simulink model "simulink"  (R2015a)
settings: Solver=ode4  StartTime=0.0  StopTime=inf  FixedStep=1e-3  RelTol=1e-3
values from neighbouring files (symbols this model uses):
  b_end1 = 0.5*(k_end1*Cyl1.m)^0.5    [m-script.m]
  b_end2 = 0.5*(k_end2*Cyl2.m)^0.5    [m-script.m]
  b_end3 = 0.5*(k_end3*Cyl3.m)^0.5    [m-script.m]
  b_end4 = 0.5*(k_end4*Cyl4.m)^0.5    [m-script.m]
  Cyl1_b = 40000    [m-script.m]
  Cyl1_Fc = 20514    [m-script.m]
  Cyl1_Fs = 22360    [m-script.m]
  Cyl1_K = 20000    [m-script.m]
  Cyl1_vs = 0.8    [m-script.m]
  Cyl2_b = 30000    [m-script.m]
  Cyl2_Fc = 14950    [m-script.m]
  Cyl2_Fs = 16125    [m-script.m]
  Cyl2_K = 20000    [m-script.m]
  Cyl2_vs = 0.8    [m-script.m]
  Cyl3_b = 30000    [m-script.m]
  Cyl3_Fc = 14996    [m-script.m]
  Cyl3_Fs = 16340    [m-script.m]
  Cyl3_K = 20000    [m-script.m]
  Cyl3_vs = 0.8    [m-script.m]
  Cyl4_b = 8500    [m-script.m]
  Cyl4_Fc = 4570    [m-script.m]
  Cyl4_Fs = 4945    [m-script.m]
  Cyl4_K = 20000    [m-script.m]
  Cyl4_vs = 0.8    [m-script.m]
  k_end1 = (pr_Ps*Cyl1.A_A)/v1    [m-script.m]
  k_end2 = (pr_Ps*Cyl2.A_A)/v2    [m-script.m]
  k_end3 = (pr_Ps*Cyl3.A_A)/v3    [m-script.m]
  k_end4 = (pr_Ps*Cyl4.A_A)/v4    [m-script.m]
  pr_Ps = 215e5    (= 21500000)    [m-script.m]
  sampleTime = 0.001    [m-script.m]
  Valve_eta = 0.989    [m-script.m]
  Valve_omega = 40.5    [m-script.m]
undefined symbols (not defined in the file or in its folder): Cyl, Cyl1, Cyl2, Cyl3, Cyl4, Cylinder2, Cylinder3, Cylinder4, Extention1, Extention2, Lift, Link1, Pillar, Pinion, Piston2, Piston3, Piston4, Rack, Tilt, Valve, X, Y, Z
undefined symbols (not defined in the file): Valve1, Valve2, Valve3, Valve4
libraries: sm_lib x72, simulink x32, nesl_utility x20, simulink_extras x3, xpcrtudplib x2, xpcobsoletelib x2
(part 4 of 4)

== system simulink/Hydraulics/Cylinder 5/Cylinder/Chamber A ==
  Q_in : Inport
  " dv_A/dt" : Inport  Port=2
  " V_A" : Inport  Port=3
  " B" : Inport  Port=4
  Integrator : Integrator  InitialCondition=pinitial  AbsoluteTolerance=10
  Product : Product  Inputs=*/*  SaturateOnIntegerOverflow=on  InputSameDT=on  OutDataTypeStr=Inherit: Same as first input
  Saturation : Saturate  UpperLimit=inf  LowerLimit=0
  Sum : Sum  Inputs=+-  SaturateOnIntegerOverflow=on  InputSameDT=on  OutDataTypeStr=Inherit: Same as first input
  p_A : Outport
  wires:
  " V_A"/1 -> Product/2
  " dv_A/dt"/1 -> Sum/2
  Product/1 -> Integrator/1
  Integrator/1 -> Saturation/1
  Saturation/1 -> p_A/1
  " B"/1 -> Product/3
  Q_in/1 -> Sum/1
  Sum/1 -> Product/1

== system simulink/Hydraulics/Cylinder 5/Cylinder/Chamber B ==
  B : Inport
  V_B : Inport  Port=2
  dv_B/dt : Inport  Port=3
  Q_in : Inport  Port=4
  Integrator : Integrator  InitialCondition=pinitial  AbsoluteTolerance=10
  Product : Product  Inputs=*/*  SaturateOnIntegerOverflow=on  InputSameDT=on  OutDataTypeStr=Inherit: Same as first input
  Saturation : Saturate  UpperLimit=inf  LowerLimit=0
  Sum : Sum  Inputs=+-  SaturateOnIntegerOverflow=on  InputSameDT=on  OutDataTypeStr=Inherit: Same as first input
  p_B : Outport
  wires:
  V_B/1 -> Product/2
  dv_B/dt/1 -> Sum/2
  Sum/1 -> Product/1
  Q_in/1 -> Sum/1
  B/1 -> Product/3
  Saturation/1 -> p_B/1
  Integrator/1 -> Saturation/1
  Product/1 -> Integrator/1

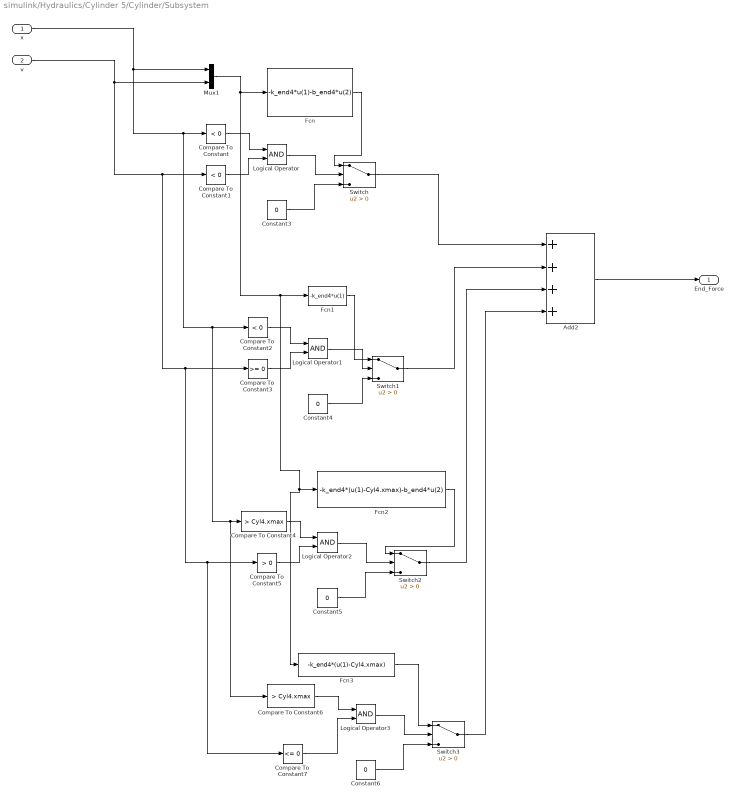
== system simulink/Hydraulics/Cylinder 5/Cylinder/Subsystem ==
  x : Inport
  v : Inport  Port=2
  Add2 : Sum  Inputs=++++
  Compare To Constant : simulink/Logic and Bit Operations/Compare To Constant  relop=<  const=0  OutDataTypeStr=boolean
  Compare To Constant1 : simulink/Logic and Bit Operations/Compare To Constant  relop=<  const=0  OutDataTypeStr=boolean
  Compare To Constant2 : simulink/Logic and Bit Operations/Compare To Constant  relop=<  const=0  OutDataTypeStr=boolean
  Compare To Constant3 : simulink/Logic and Bit Operations/Compare To Constant  relop=>=  const=0  OutDataTypeStr=boolean
  Compare To Constant4 : simulink/Logic and Bit Operations/Compare To Constant  relop=>  const=Cyl4.xmax  OutDataTypeStr=boolean
  Compare To Constant5 : simulink/Logic and Bit Operations/Compare To Constant  relop=>  const=0  OutDataTypeStr=boolean
  Compare To Constant6 : simulink/Logic and Bit Operations/Compare To Constant  relop=>  const=Cyl4.xmax  OutDataTypeStr=boolean
  Compare To Constant7 : simulink/Logic and Bit Operations/Compare To Constant  relop=<=  const=0  OutDataTypeStr=boolean
  Constant{3..6} (4 alike) : Constant  Value=0
  Fcn : Fcn  Expr=-k_end4*u(1)-b_end4*u(2)
  Fcn1 : Fcn  Expr=-k_end4*u(1)
  Fcn2 : Fcn  Expr=-k_end4*(u(1)-Cyl4.xmax)-b_end4*u(2)
  Fcn3 : Fcn  Expr=-k_end4*(u(1)-Cyl4.xmax)
  Logical Operator{,1..3} (4 alike) : Logic  AllPortsSameDT=off  OutDataTypeStr=boolean
  Mux1 : Mux  Inputs=2
  Switch{,1..3} (4 alike) : Switch  Criteria=u2 > Threshold
  End_Force : Outport
  wires:
  x/1 -> Compare To Constant/1, Compare To Constant2/1, Compare To Constant6/1, Compare To Constant4/1, Mux1/1
  v/1 -> Mux1/2, Compare To Constant1/1, Compare To Constant3/1, Compare To Constant5/1, Compare To Constant7/1
  Fcn2/1 -> Switch2/1
  Logical Operator3/1 -> Switch3/2
  Fcn3/1 -> Switch3/1
  Compare To Constant5/1 -> Logical Operator2/2
  Constant6/1 -> Switch3/3
  Switch2/1 -> Add2/3
  Compare To Constant6/1 -> Logical Operator3/1
  Switch/1 -> Add2/1
  Logical Operator2/1 -> Switch2/2
  Compare To Constant7/1 -> Logical Operator3/2
  Switch1/1 -> Add2/2
  Add2/1 -> End_Force/1
  Mux1/1 -> Fcn1/1, Fcn2/1, Fcn3/1, Fcn/1
  Switch3/1 -> Add2/4
  Compare To Constant2/1 -> Logical Operator1/1
  Compare To Constant1/1 -> Logical Operator/2
  Constant5/1 -> Switch2/3
  Constant4/1 -> Switch1/3
  Logical Operator1/1 -> Switch1/2
  Fcn/1 -> Switch/1
  Logical Operator/1 -> Switch/2
  Constant3/1 -> Switch/3
  Compare To Constant/1 -> Logical Operator/1
  Compare To Constant4/1 -> Logical Operator2/1
  Fcn1/1 -> Switch1/1
  Compare To Constant3/1 -> Logical Operator1/2

== system simulink/Hydraulics/Cylinder 1/4//3 Valve/Flow paths/Orifice AT ==
  p_A : Inport
  p_T : Inport  Port=2
  u : Inport  Port=3
  Abs : Abs  ZeroCross=off  SaturateOnIntegerOverflow=on
  Add : Sum  Inputs=+-
  Fcn : Fcn  Expr=u[2]*u[1]/2.0/sqrt(ptr)*(3-u[1]/ptr)
  Fcn-Saturation : Fcn  Expr=(u(1)>=-1e-10)*u(1)
  Gain : Gain  Gain=K  SaturateOnIntegerOverflow=on  OutDataTypeStr=Inherit: Same as input  ParamDataTypeStr=Inherit: Same as input
  Gain1 : Gain  Gain=-1  SaturateOnIntegerOverflow=on  OutDataTypeStr=Inherit: Same as input  ParamDataTypeStr=Inherit: Same as input
  Math Function1 : Math  Operator=sqrt  SaturateOnIntegerOverflow=on
  Mux : Mux  Inputs=2
  Product : Product  SaturateOnIntegerOverflow=on  InputSameDT=on  OutDataTypeStr=Inherit: Same as first input
  Product1 : Product  SaturateOnIntegerOverflow=on  InputSameDT=on  OutDataTypeStr=Inherit: Same as first input
  Sign : Signum  ZeroCross=off
  "Switch, treshold = ptr" : Switch  Threshold=ptr  ZeroCross=off  SaturateOnIntegerOverflow=on
  Q_A : Outport  InitialOutput=0
  Q_T : Outport  Port=2  InitialOutput=0
  wires:
  u/1 -> Fcn-Saturation/1
  Fcn/1 -> "Switch, treshold = ptr"/3
  Mux/1 -> Fcn/1
  Product/1 -> "Switch, treshold = ptr"/1
  Math Function1/1 -> Product/1
  Abs/1 -> "Switch, treshold = ptr"/2, Mux/1, Math Function1/1
  Fcn-Saturation/1 -> Gain/1
  Gain/1 -> Product/2, Mux/2
  "Switch, treshold = ptr"/1 -> Product1/2
  Sign/1 -> Product1/1
  p_A/1 -> Add/1
  p_T/1 -> Add/2
  Add/1 -> Abs/1, Sign/1
  Product1/1 -> Q_T/1, Gain1/1
  Gain1/1 -> Q_A/1

== system simulink/Hydraulics/Cylinder 1/4//3 Valve/Flow paths/Orifice BT ==
  p_T : Inport
  p_B : Inport  Port=2
  u : Inport  Port=3
  Abs : Abs  ZeroCross=off  SaturateOnIntegerOverflow=on
  Add : Sum  Inputs=+-
  Fcn : Fcn  Expr=u[2]*u[1]/2.0/sqrt(ptr)*(3-u[1]/ptr)
  Fcn-Saturation : Fcn  Expr=(u(1)>=-1e-10)*u(1)
  Gain : Gain  Gain=K  SaturateOnIntegerOverflow=on  OutDataTypeStr=Inherit: Same as input  ParamDataTypeStr=Inherit: Same as input
  Gain1 : Gain  Gain=-1  SaturateOnIntegerOverflow=on  OutDataTypeStr=Inherit: Same as input  ParamDataTypeStr=Inherit: Same as input
  Math Function1 : Math  Operator=sqrt  SaturateOnIntegerOverflow=on
  Mux : Mux  Inputs=2
  Product : Product  SaturateOnIntegerOverflow=on  InputSameDT=on  OutDataTypeStr=Inherit: Same as first input
  Product1 : Product  SaturateOnIntegerOverflow=on  InputSameDT=on  OutDataTypeStr=Inherit: Same as first input
  Sign : Signum  ZeroCross=off
  "Switch, treshold = ptr" : Switch  Threshold=ptr  ZeroCross=off  SaturateOnIntegerOverflow=on
  Q_T : Outport  InitialOutput=0
  Q_B : Outport  Port=2  InitialOutput=0
  wires:
  Gain1/1 -> Q_T/1
  Product1/1 -> Gain1/1, Q_B/1
  Add/1 -> Sign/1, Abs/1
  p_B/1 -> Add/2
  p_T/1 -> Add/1
  Sign/1 -> Product1/1
  "Switch, treshold = ptr"/1 -> Product1/2
  Gain/1 -> Mux/2, Product/2
  Fcn-Saturation/1 -> Gain/1
  Abs/1 -> Math Function1/1, Mux/1, "Switch, treshold = ptr"/2
  Math Function1/1 -> Product/1
  Product/1 -> "Switch, treshold = ptr"/1
  Mux/1 -> Fcn/1
  Fcn/1 -> "Switch, treshold = ptr"/3
  u/1 -> Fcn-Saturation/1

== system simulink/Hydraulics/Cylinder 1/4//3 Valve/Flow paths/Orifice PA ==
  p_P : Inport
  p_A : Inport  Port=2
  u : Inport  Port=3
  Abs : Abs  ZeroCross=off  SaturateOnIntegerOverflow=on
  Add : Sum  Inputs=+-
  Fcn : Fcn  Expr=u[2]*u[1]/2.0/sqrt(ptr)*(3-u[1]/ptr)
  Fcn-Saturation : Fcn  Expr=(u(1)>=-1e-10)*u(1)
  Gain : Gain  Gain=K  SaturateOnIntegerOverflow=on  OutDataTypeStr=Inherit: Same as input  ParamDataTypeStr=Inherit: Same as input
  Gain1 : Gain  Gain=-1  SaturateOnIntegerOverflow=on  OutDataTypeStr=Inherit: Same as input  ParamDataTypeStr=Inherit: Same as input
  Math Function1 : Math  Operator=sqrt  SaturateOnIntegerOverflow=on
  Mux : Mux  Inputs=2
  Product : Product  SaturateOnIntegerOverflow=on  InputSameDT=on  OutDataTypeStr=Inherit: Same as first input
  Product1 : Product  SaturateOnIntegerOverflow=on  InputSameDT=on  OutDataTypeStr=Inherit: Same as first input
  Sign : Signum  ZeroCross=off
  "Switch, treshold = ptr" : Switch  Threshold=ptr  ZeroCross=off  SaturateOnIntegerOverflow=on
  Q_P : Outport  InitialOutput=0
  Q_A : Outport  Port=2  InitialOutput=0
  wires:
  u/1 -> Fcn-Saturation/1
  Fcn/1 -> "Switch, treshold = ptr"/3
  Mux/1 -> Fcn/1
  Product/1 -> "Switch, treshold = ptr"/1
  Math Function1/1 -> Product/1
  Abs/1 -> "Switch, treshold = ptr"/2, Mux/1, Math Function1/1
  Fcn-Saturation/1 -> Gain/1
  Gain/1 -> Product/2, Mux/2
  "Switch, treshold = ptr"/1 -> Product1/2
  Sign/1 -> Product1/1
  p_P/1 -> Add/1
  p_A/1 -> Add/2
  Add/1 -> Abs/1, Sign/1
  Product1/1 -> Q_A/1, Gain1/1
  Gain1/1 -> Q_P/1

== system simulink/Hydraulics/Cylinder 1/4//3 Valve/Flow paths/Orifice PB ==
  p_B : Inport
  p_P : Inport  Port=2
  u : Inport  Port=3
  Abs : Abs  ZeroCross=off  SaturateOnIntegerOverflow=on
  Add : Sum  Inputs=+-
  Fcn : Fcn  Expr=u[2]*u[1]/2.0/sqrt(ptr)*(3-u[1]/ptr)
  Fcn-Saturation : Fcn  Expr=(u(1)>=-1e-10)*u(1)
  Gain : Gain  Gain=K  SaturateOnIntegerOverflow=on  OutDataTypeStr=Inherit: Same as input  ParamDataTypeStr=Inherit: Same as input
  Gain1 : Gain  Gain=-1  SaturateOnIntegerOverflow=on  OutDataTypeStr=Inherit: Same as input  ParamDataTypeStr=Inherit: Same as input
  Math Function1 : Math  Operator=sqrt  SaturateOnIntegerOverflow=on
  Mux : Mux  Inputs=2
  Product : Product  SaturateOnIntegerOverflow=on  InputSameDT=on  OutDataTypeStr=Inherit: Same as first input
  Product1 : Product  SaturateOnIntegerOverflow=on  InputSameDT=on  OutDataTypeStr=Inherit: Same as first input
  Sign : Signum  ZeroCross=off
  "Switch, treshold = ptr" : Switch  Threshold=ptr  ZeroCross=off  SaturateOnIntegerOverflow=on
  Q_B : Outport  InitialOutput=0
  Q_P : Outport  Port=2  InitialOutput=0
  wires:
  Gain1/1 -> Q_B/1
  Product1/1 -> Gain1/1, Q_P/1
  Add/1 -> Sign/1, Abs/1
  p_P/1 -> Add/2
  p_B/1 -> Add/1
  Sign/1 -> Product1/1
  "Switch, treshold = ptr"/1 -> Product1/2
  Gain/1 -> Mux/2, Product/2
  Fcn-Saturation/1 -> Gain/1
  Abs/1 -> Math Function1/1, Mux/1, "Switch, treshold = ptr"/2
  Math Function1/1 -> Product/1
  Product/1 -> "Switch, treshold = ptr"/1
  Mux/1 -> Fcn/1
  Fcn/1 -> "Switch, treshold = ptr"/3
  u/1 -> Fcn-Saturation/1

== system simulink/Hydraulics/Cylinder 2/4//3 Valve/Flow paths/Orifice AT ==
  p_A : Inport
  p_T : Inport  Port=2
  u : Inport  Port=3
  Abs : Abs  ZeroCross=off  SaturateOnIntegerOverflow=on
  Add : Sum  Inputs=+-
  Fcn : Fcn  Expr=u[2]*u[1]/2.0/sqrt(ptr)*(3-u[1]/ptr)
  Fcn-Saturation : Fcn  Expr=(u(1)>=-1e-10)*u(1)
  Gain : Gain  Gain=K  SaturateOnIntegerOverflow=on  OutDataTypeStr=Inherit: Same as input  ParamDataTypeStr=Inherit: Same as input
  Gain1 : Gain  Gain=-1  SaturateOnIntegerOverflow=on  OutDataTypeStr=Inherit: Same as input  ParamDataTypeStr=Inherit: Same as input
  Math Function1 : Math  Operator=sqrt  SaturateOnIntegerOverflow=on
  Mux : Mux  Inputs=2
  Product : Product  SaturateOnIntegerOverflow=on  InputSameDT=on  OutDataTypeStr=Inherit: Same as first input
  Product1 : Product  SaturateOnIntegerOverflow=on  InputSameDT=on  OutDataTypeStr=Inherit: Same as first input
  Sign : Signum  ZeroCross=off
  "Switch, treshold = ptr" : Switch  Threshold=ptr  ZeroCross=off  SaturateOnIntegerOverflow=on
  Q_A : Outport  InitialOutput=0
  Q_T : Outport  Port=2  InitialOutput=0
  wires:
  u/1 -> Fcn-Saturation/1
  Fcn/1 -> "Switch, treshold = ptr"/3
  Mux/1 -> Fcn/1
  Product/1 -> "Switch, treshold = ptr"/1
  Math Function1/1 -> Product/1
  Abs/1 -> "Switch, treshold = ptr"/2, Mux/1, Math Function1/1
  Fcn-Saturation/1 -> Gain/1
  Gain/1 -> Product/2, Mux/2
  "Switch, treshold = ptr"/1 -> Product1/2
  Sign/1 -> Product1/1
  p_A/1 -> Add/1
  p_T/1 -> Add/2
  Add/1 -> Abs/1, Sign/1
  Product1/1 -> Q_T/1, Gain1/1
  Gain1/1 -> Q_A/1

== system simulink/Hydraulics/Cylinder 2/4//3 Valve/Flow paths/Orifice BT ==
  p_T : Inport
  p_B : Inport  Port=2
  u : Inport  Port=3
  Abs : Abs  ZeroCross=off  SaturateOnIntegerOverflow=on
  Add : Sum  Inputs=+-
  Fcn : Fcn  Expr=u[2]*u[1]/2.0/sqrt(ptr)*(3-u[1]/ptr)
  Fcn-Saturation : Fcn  Expr=(u(1)>=-1e-10)*u(1)
  Gain : Gain  Gain=K  SaturateOnIntegerOverflow=on  OutDataTypeStr=Inherit: Same as input  ParamDataTypeStr=Inherit: Same as input
  Gain1 : Gain  Gain=-1  SaturateOnIntegerOverflow=on  OutDataTypeStr=Inherit: Same as input  ParamDataTypeStr=Inherit: Same as input
  Math Function1 : Math  Operator=sqrt  SaturateOnIntegerOverflow=on
  Mux : Mux  Inputs=2
  Product : Product  SaturateOnIntegerOverflow=on  InputSameDT=on  OutDataTypeStr=Inherit: Same as first input
  Product1 : Product  SaturateOnIntegerOverflow=on  InputSameDT=on  OutDataTypeStr=Inherit: Same as first input
  Sign : Signum  ZeroCross=off
  "Switch, treshold = ptr" : Switch  Threshold=ptr  ZeroCross=off  SaturateOnIntegerOverflow=on
  Q_T : Outport  InitialOutput=0
  Q_B : Outport  Port=2  InitialOutput=0
  wires:
  Gain1/1 -> Q_T/1
  Product1/1 -> Gain1/1, Q_B/1
  Add/1 -> Sign/1, Abs/1
  p_B/1 -> Add/2
  p_T/1 -> Add/1
  Sign/1 -> Product1/1
  "Switch, treshold = ptr"/1 -> Product1/2
  Gain/1 -> Mux/2, Product/2
  Fcn-Saturation/1 -> Gain/1
  Abs/1 -> Math Function1/1, Mux/1, "Switch, treshold = ptr"/2
  Math Function1/1 -> Product/1
  Product/1 -> "Switch, treshold = ptr"/1
  Mux/1 -> Fcn/1
  Fcn/1 -> "Switch, treshold = ptr"/3
  u/1 -> Fcn-Saturation/1

== system simulink/Hydraulics/Cylinder 2/4//3 Valve/Flow paths/Orifice PA ==
  p_P : Inport
  p_A : Inport  Port=2
  u : Inport  Port=3
  Abs : Abs  ZeroCross=off  SaturateOnIntegerOverflow=on
  Add : Sum  Inputs=+-
  Fcn : Fcn  Expr=u[2]*u[1]/2.0/sqrt(ptr)*(3-u[1]/ptr)
  Fcn-Saturation : Fcn  Expr=(u(1)>=-1e-10)*u(1)
  Gain : Gain  Gain=K  SaturateOnIntegerOverflow=on  OutDataTypeStr=Inherit: Same as input  ParamDataTypeStr=Inherit: Same as input
  Gain1 : Gain  Gain=-1  SaturateOnIntegerOverflow=on  OutDataTypeStr=Inherit: Same as input  ParamDataTypeStr=Inherit: Same as input
  Math Function1 : Math  Operator=sqrt  SaturateOnIntegerOverflow=on
  Mux : Mux  Inputs=2
  Product : Product  SaturateOnIntegerOverflow=on  InputSameDT=on  OutDataTypeStr=Inherit: Same as first input
  Product1 : Product  SaturateOnIntegerOverflow=on  InputSameDT=on  OutDataTypeStr=Inherit: Same as first input
  Sign : Signum  ZeroCross=off
  "Switch, treshold = ptr" : Switch  Threshold=ptr  ZeroCross=off  SaturateOnIntegerOverflow=on
  Q_P : Outport  InitialOutput=0
  Q_A : Outport  Port=2  InitialOutput=0
  wires:
  u/1 -> Fcn-Saturation/1
  Fcn/1 -> "Switch, treshold = ptr"/3
  Mux/1 -> Fcn/1
  Product/1 -> "Switch, treshold = ptr"/1
  Math Function1/1 -> Product/1
  Abs/1 -> "Switch, treshold = ptr"/2, Mux/1, Math Function1/1
  Fcn-Saturation/1 -> Gain/1
  Gain/1 -> Product/2, Mux/2
  "Switch, treshold = ptr"/1 -> Product1/2
  Sign/1 -> Product1/1
  p_P/1 -> Add/1
  p_A/1 -> Add/2
  Add/1 -> Abs/1, Sign/1
  Product1/1 -> Q_A/1, Gain1/1
  Gain1/1 -> Q_P/1

== system simulink/Hydraulics/Cylinder 2/4//3 Valve/Flow paths/Orifice PB ==
  p_B : Inport
  p_P : Inport  Port=2
  u : Inport  Port=3
  Abs : Abs  ZeroCross=off  SaturateOnIntegerOverflow=on
  Add : Sum  Inputs=+-
  Fcn : Fcn  Expr=u[2]*u[1]/2.0/sqrt(ptr)*(3-u[1]/ptr)
  Fcn-Saturation : Fcn  Expr=(u(1)>=-1e-10)*u(1)
  Gain : Gain  Gain=K  SaturateOnIntegerOverflow=on  OutDataTypeStr=Inherit: Same as input  ParamDataTypeStr=Inherit: Same as input
  Gain1 : Gain  Gain=-1  SaturateOnIntegerOverflow=on  OutDataTypeStr=Inherit: Same as input  ParamDataTypeStr=Inherit: Same as input
  Math Function1 : Math  Operator=sqrt  SaturateOnIntegerOverflow=on
  Mux : Mux  Inputs=2
  Product : Product  SaturateOnIntegerOverflow=on  InputSameDT=on  OutDataTypeStr=Inherit: Same as first input
  Product1 : Product  SaturateOnIntegerOverflow=on  InputSameDT=on  OutDataTypeStr=Inherit: Same as first input
  Sign : Signum  ZeroCross=off
  "Switch, treshold = ptr" : Switch  Threshold=ptr  ZeroCross=off  SaturateOnIntegerOverflow=on
  Q_B : Outport  InitialOutput=0
  Q_P : Outport  Port=2  InitialOutput=0
  wires:
  Gain1/1 -> Q_B/1
  Product1/1 -> Gain1/1, Q_P/1
  Add/1 -> Sign/1, Abs/1
  p_P/1 -> Add/2
  p_B/1 -> Add/1
  Sign/1 -> Product1/1
  "Switch, treshold = ptr"/1 -> Product1/2
  Gain/1 -> Mux/2, Product/2
  Fcn-Saturation/1 -> Gain/1
  Abs/1 -> Math Function1/1, Mux/1, "Switch, treshold = ptr"/2
  Math Function1/1 -> Product/1
  Product/1 -> "Switch, treshold = ptr"/1
  Mux/1 -> Fcn/1
  Fcn/1 -> "Switch, treshold = ptr"/3
  u/1 -> Fcn-Saturation/1

== system simulink/Hydraulics/Cylinder 3/4//3 Valve/Flow paths/Orifice AT ==
  p_A : Inport
  p_T : Inport  Port=2
  u : Inport  Port=3
  Abs : Abs  ZeroCross=off  SaturateOnIntegerOverflow=on
  Add : Sum  Inputs=+-
  Fcn : Fcn  Expr=u[2]*u[1]/2.0/sqrt(ptr)*(3-u[1]/ptr)
  Fcn-Saturation : Fcn  Expr=(u(1)>=-1e-10)*u(1)
  Gain : Gain  Gain=K  SaturateOnIntegerOverflow=on  OutDataTypeStr=Inherit: Same as input  ParamDataTypeStr=Inherit: Same as input
  Gain1 : Gain  Gain=-1  SaturateOnIntegerOverflow=on  OutDataTypeStr=Inherit: Same as input  ParamDataTypeStr=Inherit: Same as input
  Math Function1 : Math  Operator=sqrt  SaturateOnIntegerOverflow=on
  Mux : Mux  Inputs=2
  Product : Product  SaturateOnIntegerOverflow=on  InputSameDT=on  OutDataTypeStr=Inherit: Same as first input
  Product1 : Product  SaturateOnIntegerOverflow=on  InputSameDT=on  OutDataTypeStr=Inherit: Same as first input
  Sign : Signum  ZeroCross=off
  "Switch, treshold = ptr" : Switch  Threshold=ptr  ZeroCross=off  SaturateOnIntegerOverflow=on
  Q_A : Outport  InitialOutput=0
  Q_T : Outport  Port=2  InitialOutput=0
  wires:
  u/1 -> Fcn-Saturation/1
  Fcn/1 -> "Switch, treshold = ptr"/3
  Mux/1 -> Fcn/1
  Product/1 -> "Switch, treshold = ptr"/1
  Math Function1/1 -> Product/1
  Abs/1 -> "Switch, treshold = ptr"/2, Mux/1, Math Function1/1
  Fcn-Saturation/1 -> Gain/1
  Gain/1 -> Product/2, Mux/2
  "Switch, treshold = ptr"/1 -> Product1/2
  Sign/1 -> Product1/1
  p_A/1 -> Add/1
  p_T/1 -> Add/2
  Add/1 -> Abs/1, Sign/1
  Product1/1 -> Q_T/1, Gain1/1
  Gain1/1 -> Q_A/1

== system simulink/Hydraulics/Cylinder 3/4//3 Valve/Flow paths/Orifice BT ==
  p_T : Inport
  p_B : Inport  Port=2
  u : Inport  Port=3
  Abs : Abs  ZeroCross=off  SaturateOnIntegerOverflow=on
  Add : Sum  Inputs=+-
  Fcn : Fcn  Expr=u[2]*u[1]/2.0/sqrt(ptr)*(3-u[1]/ptr)
  Fcn-Saturation : Fcn  Expr=(u(1)>=-1e-10)*u(1)
  Gain : Gain  Gain=K  SaturateOnIntegerOverflow=on  OutDataTypeStr=Inherit: Same as input  ParamDataTypeStr=Inherit: Same as input
  Gain1 : Gain  Gain=-1  SaturateOnIntegerOverflow=on  OutDataTypeStr=Inherit: Same as input  ParamDataTypeStr=Inherit: Same as input
  Math Function1 : Math  Operator=sqrt  SaturateOnIntegerOverflow=on
  Mux : Mux  Inputs=2
  Product : Product  SaturateOnIntegerOverflow=on  InputSameDT=on  OutDataTypeStr=Inherit: Same as first input
  Product1 : Product  SaturateOnIntegerOverflow=on  InputSameDT=on  OutDataTypeStr=Inherit: Same as first input
  Sign : Signum  ZeroCross=off
  "Switch, treshold = ptr" : Switch  Threshold=ptr  ZeroCross=off  SaturateOnIntegerOverflow=on
  Q_T : Outport  InitialOutput=0
  Q_B : Outport  Port=2  InitialOutput=0
  wires:
  Gain1/1 -> Q_T/1
  Product1/1 -> Gain1/1, Q_B/1
  Add/1 -> Sign/1, Abs/1
  p_B/1 -> Add/2
  p_T/1 -> Add/1
  Sign/1 -> Product1/1
  "Switch, treshold = ptr"/1 -> Product1/2
  Gain/1 -> Mux/2, Product/2
  Fcn-Saturation/1 -> Gain/1
  Abs/1 -> Math Function1/1, Mux/1, "Switch, treshold = ptr"/2
  Math Function1/1 -> Product/1
  Product/1 -> "Switch, treshold = ptr"/1
  Mux/1 -> Fcn/1
  Fcn/1 -> "Switch, treshold = ptr"/3
  u/1 -> Fcn-Saturation/1

== system simulink/Hydraulics/Cylinder 3/4//3 Valve/Flow paths/Orifice PA ==
  p_P : Inport
  p_A : Inport  Port=2
  u : Inport  Port=3
  Abs : Abs  ZeroCross=off  SaturateOnIntegerOverflow=on
  Add : Sum  Inputs=+-
  Fcn : Fcn  Expr=u[2]*u[1]/2.0/sqrt(ptr)*(3-u[1]/ptr)
  Fcn-Saturation : Fcn  Expr=(u(1)>=-1e-10)*u(1)
  Gain : Gain  Gain=K  SaturateOnIntegerOverflow=on  OutDataTypeStr=Inherit: Same as input  ParamDataTypeStr=Inherit: Same as input
  Gain1 : Gain  Gain=-1  SaturateOnIntegerOverflow=on  OutDataTypeStr=Inherit: Same as input  ParamDataTypeStr=Inherit: Same as input
  Math Function1 : Math  Operator=sqrt  SaturateOnIntegerOverflow=on
  Mux : Mux  Inputs=2
  Product : Product  SaturateOnIntegerOverflow=on  InputSameDT=on  OutDataTypeStr=Inherit: Same as first input
  Product1 : Product  SaturateOnIntegerOverflow=on  InputSameDT=on  OutDataTypeStr=Inherit: Same as first input
  Sign : Signum  ZeroCross=off
  "Switch, treshold = ptr" : Switch  Threshold=ptr  ZeroCross=off  SaturateOnIntegerOverflow=on
  Q_P : Outport  InitialOutput=0
  Q_A : Outport  Port=2  InitialOutput=0
  wires:
  u/1 -> Fcn-Saturation/1
  Fcn/1 -> "Switch, treshold = ptr"/3
  Mux/1 -> Fcn/1
  Product/1 -> "Switch, treshold = ptr"/1
  Math Function1/1 -> Product/1
  Abs/1 -> "Switch, treshold = ptr"/2, Mux/1, Math Function1/1
  Fcn-Saturation/1 -> Gain/1
  Gain/1 -> Product/2, Mux/2
  "Switch, treshold = ptr"/1 -> Product1/2
  Sign/1 -> Product1/1
  p_P/1 -> Add/1
  p_A/1 -> Add/2
  Add/1 -> Abs/1, Sign/1
  Product1/1 -> Q_A/1, Gain1/1
  Gain1/1 -> Q_P/1

== system simulink/Hydraulics/Cylinder 3/4//3 Valve/Flow paths/Orifice PB ==
  p_B : Inport
  p_P : Inport  Port=2
  u : Inport  Port=3
  Abs : Abs  ZeroCross=off  SaturateOnIntegerOverflow=on
  Add : Sum  Inputs=+-
  Fcn : Fcn  Expr=u[2]*u[1]/2.0/sqrt(ptr)*(3-u[1]/ptr)
  Fcn-Saturation : Fcn  Expr=(u(1)>=-1e-10)*u(1)
  Gain : Gain  Gain=K  SaturateOnIntegerOverflow=on  OutDataTypeStr=Inherit: Same as input  ParamDataTypeStr=Inherit: Same as input
  Gain1 : Gain  Gain=-1  SaturateOnIntegerOverflow=on  OutDataTypeStr=Inherit: Same as input  ParamDataTypeStr=Inherit: Same as input
  Math Function1 : Math  Operator=sqrt  SaturateOnIntegerOverflow=on
  Mux : Mux  Inputs=2
  Product : Product  SaturateOnIntegerOverflow=on  InputSameDT=on  OutDataTypeStr=Inherit: Same as first input
  Product1 : Product  SaturateOnIntegerOverflow=on  InputSameDT=on  OutDataTypeStr=Inherit: Same as first input
  Sign : Signum  ZeroCross=off
  "Switch, treshold = ptr" : Switch  Threshold=ptr  ZeroCross=off  SaturateOnIntegerOverflow=on
  Q_B : Outport  InitialOutput=0
  Q_P : Outport  Port=2  InitialOutput=0
  wires:
  Gain1/1 -> Q_B/1
  Product1/1 -> Gain1/1, Q_P/1
  Add/1 -> Sign/1, Abs/1
  p_P/1 -> Add/2
  p_B/1 -> Add/1
  Sign/1 -> Product1/1
  "Switch, treshold = ptr"/1 -> Product1/2
  Gain/1 -> Mux/2, Product/2
  Fcn-Saturation/1 -> Gain/1
  Abs/1 -> Math Function1/1, Mux/1, "Switch, treshold = ptr"/2
  Math Function1/1 -> Product/1
  Product/1 -> "Switch, treshold = ptr"/1
  Mux/1 -> Fcn/1
  Fcn/1 -> "Switch, treshold = ptr"/3
  u/1 -> Fcn-Saturation/1

== system simulink/Hydraulics/Cylinder 5/4//3 Valve/Flow paths/Orifice AT ==
  p_A : Inport
  p_T : Inport  Port=2
  u : Inport  Port=3
  Abs : Abs  ZeroCross=off  SaturateOnIntegerOverflow=on
  Add : Sum  Inputs=+-
  Fcn : Fcn  Expr=u[2]*u[1]/2.0/sqrt(ptr)*(3-u[1]/ptr)
  Fcn-Saturation : Fcn  Expr=(u(1)>=-1e-10)*u(1)
  Gain : Gain  Gain=K  SaturateOnIntegerOverflow=on  OutDataTypeStr=Inherit: Same as input  ParamDataTypeStr=Inherit: Same as input
  Gain1 : Gain  Gain=-1  SaturateOnIntegerOverflow=on  OutDataTypeStr=Inherit: Same as input  ParamDataTypeStr=Inherit: Same as input
  Math Function1 : Math  Operator=sqrt  SaturateOnIntegerOverflow=on
  Mux : Mux  Inputs=2
  Product : Product  SaturateOnIntegerOverflow=on  InputSameDT=on  OutDataTypeStr=Inherit: Same as first input
  Product1 : Product  SaturateOnIntegerOverflow=on  InputSameDT=on  OutDataTypeStr=Inherit: Same as first input
  Sign : Signum  ZeroCross=off
  "Switch, treshold = ptr" : Switch  Threshold=ptr  ZeroCross=off  SaturateOnIntegerOverflow=on
  Q_A : Outport  InitialOutput=0
  Q_T : Outport  Port=2  InitialOutput=0
  wires:
  Gain1/1 -> Q_A/1
  Product1/1 -> Gain1/1, Q_T/1
  Add/1 -> Sign/1, Abs/1
  p_T/1 -> Add/2
  p_A/1 -> Add/1
  Sign/1 -> Product1/1
  "Switch, treshold = ptr"/1 -> Product1/2
  Gain/1 -> Mux/2, Product/2
  Fcn-Saturation/1 -> Gain/1
  Abs/1 -> Math Function1/1, Mux/1, "Switch, treshold = ptr"/2
  Math Function1/1 -> Product/1
  Product/1 -> "Switch, treshold = ptr"/1
  Mux/1 -> Fcn/1
  Fcn/1 -> "Switch, treshold = ptr"/3
  u/1 -> Fcn-Saturation/1

== system simulink/Hydraulics/Cylinder 5/4//3 Valve/Flow paths/Orifice BT ==
  p_T : Inport
  p_B : Inport  Port=2
  u : Inport  Port=3
  Abs : Abs  ZeroCross=off  SaturateOnIntegerOverflow=on
  Add : Sum  Inputs=+-
  Fcn : Fcn  Expr=u[2]*u[1]/2.0/sqrt(ptr)*(3-u[1]/ptr)
  Fcn-Saturation : Fcn  Expr=(u(1)>=-1e-10)*u(1)
  Gain : Gain  Gain=K  SaturateOnIntegerOverflow=on  OutDataTypeStr=Inherit: Same as input  ParamDataTypeStr=Inherit: Same as input
  Gain1 : Gain  Gain=-1  SaturateOnIntegerOverflow=on  OutDataTypeStr=Inherit: Same as input  ParamDataTypeStr=Inherit: Same as input
  Math Function1 : Math  Operator=sqrt  SaturateOnIntegerOverflow=on
  Mux : Mux  Inputs=2
  Product : Product  SaturateOnIntegerOverflow=on  InputSameDT=on  OutDataTypeStr=Inherit: Same as first input
  Product1 : Product  SaturateOnIntegerOverflow=on  InputSameDT=on  OutDataTypeStr=Inherit: Same as first input
  Sign : Signum  ZeroCross=off
  "Switch, treshold = ptr" : Switch  Threshold=ptr  ZeroCross=off  SaturateOnIntegerOverflow=on
  Q_T : Outport  InitialOutput=0
  Q_B : Outport  Port=2  InitialOutput=0
  wires:
  u/1 -> Fcn-Saturation/1
  Fcn/1 -> "Switch, treshold = ptr"/3
  Mux/1 -> Fcn/1
  Product/1 -> "Switch, treshold = ptr"/1
  Math Function1/1 -> Product/1
  Abs/1 -> "Switch, treshold = ptr"/2, Mux/1, Math Function1/1
  Fcn-Saturation/1 -> Gain/1
  Gain/1 -> Product/2, Mux/2
  "Switch, treshold = ptr"/1 -> Product1/2
  Sign/1 -> Product1/1
  p_T/1 -> Add/1
  p_B/1 -> Add/2
  Add/1 -> Abs/1, Sign/1
  Product1/1 -> Q_B/1, Gain1/1
  Gain1/1 -> Q_T/1

== system simulink/Hydraulics/Cylinder 5/4//3 Valve/Flow paths/Orifice PA ==
  p_P : Inport
  p_A : Inport  Port=2
  u : Inport  Port=3
  Abs : Abs  ZeroCross=off  SaturateOnIntegerOverflow=on
  Add : Sum  Inputs=+-
  Fcn : Fcn  Expr=u[2]*u[1]/2.0/sqrt(ptr)*(3-u[1]/ptr)
  Fcn-Saturation : Fcn  Expr=(u(1)>=-1e-10)*u(1)
  Gain : Gain  Gain=K  SaturateOnIntegerOverflow=on  OutDataTypeStr=Inherit: Same as input  ParamDataTypeStr=Inherit: Same as input
  Gain1 : Gain  Gain=-1  SaturateOnIntegerOverflow=on  OutDataTypeStr=Inherit: Same as input  ParamDataTypeStr=Inherit: Same as input
  Math Function1 : Math  Operator=sqrt  SaturateOnIntegerOverflow=on
  Mux : Mux  Inputs=2
  Product : Product  SaturateOnIntegerOverflow=on  InputSameDT=on  OutDataTypeStr=Inherit: Same as first input
  Product1 : Product  SaturateOnIntegerOverflow=on  InputSameDT=on  OutDataTypeStr=Inherit: Same as first input
  Sign : Signum  ZeroCross=off
  "Switch, treshold = ptr" : Switch  Threshold=ptr  ZeroCross=off  SaturateOnIntegerOverflow=on
  Q_P : Outport  InitialOutput=0
  Q_A : Outport  Port=2  InitialOutput=0
  wires:
  Gain1/1 -> Q_P/1
  Product1/1 -> Gain1/1, Q_A/1
  Add/1 -> Sign/1, Abs/1
  p_A/1 -> Add/2
  p_P/1 -> Add/1
  Sign/1 -> Product1/1
  "Switch, treshold = ptr"/1 -> Product1/2
  Gain/1 -> Mux/2, Product/2
  Fcn-Saturation/1 -> Gain/1
  Abs/1 -> Math Function1/1, Mux/1, "Switch, treshold = ptr"/2
  Math Function1/1 -> Product/1
  Product/1 -> "Switch, treshold = ptr"/1
  Mux/1 -> Fcn/1
  Fcn/1 -> "Switch, treshold = ptr"/3
  u/1 -> Fcn-Saturation/1

== system simulink/Hydraulics/Cylinder 5/4//3 Valve/Flow paths/Orifice PB ==
  p_B : Inport
  p_P : Inport  Port=2
  u : Inport  Port=3
  Abs : Abs  ZeroCross=off  SaturateOnIntegerOverflow=on
  Add : Sum  Inputs=+-
  Fcn : Fcn  Expr=u[2]*u[1]/2.0/sqrt(ptr)*(3-u[1]/ptr)
  Fcn-Saturation : Fcn  Expr=(u(1)>=-1e-10)*u(1)
  Gain : Gain  Gain=K  SaturateOnIntegerOverflow=on  OutDataTypeStr=Inherit: Same as input  ParamDataTypeStr=Inherit: Same as input
  Gain1 : Gain  Gain=-1  SaturateOnIntegerOverflow=on  OutDataTypeStr=Inherit: Same as input  ParamDataTypeStr=Inherit: Same as input
  Math Function1 : Math  Operator=sqrt  SaturateOnIntegerOverflow=on
  Mux : Mux  Inputs=2
  Product : Product  SaturateOnIntegerOverflow=on  InputSameDT=on  OutDataTypeStr=Inherit: Same as first input
  Product1 : Product  SaturateOnIntegerOverflow=on  InputSameDT=on  OutDataTypeStr=Inherit: Same as first input
  Sign : Signum  ZeroCross=off
  "Switch, treshold = ptr" : Switch  Threshold=ptr  ZeroCross=off  SaturateOnIntegerOverflow=on
  Q_B : Outport  InitialOutput=0
  Q_P : Outport  Port=2  InitialOutput=0
  wires:
  u/1 -> Fcn-Saturation/1
  Fcn/1 -> "Switch, treshold = ptr"/3
  Mux/1 -> Fcn/1
  Product/1 -> "Switch, treshold = ptr"/1
  Math Function1/1 -> Product/1
  Abs/1 -> "Switch, treshold = ptr"/2, Mux/1, Math Function1/1
  Fcn-Saturation/1 -> Gain/1
  Gain/1 -> Product/2, Mux/2
  "Switch, treshold = ptr"/1 -> Product1/2
  Sign/1 -> Product1/1
  p_B/1 -> Add/1
  p_P/1 -> Add/2
  Add/1 -> Abs/1, Sign/1
  Product1/1 -> Q_P/1, Gain1/1
  Gain1/1 -> Q_B/1
